simulink model "acc_aeb_top"  (R2025a)
settings: Solver=ode23t  StartTime=0.0  StopTime=40  RelTol=1e-3
undefined symbols (not defined in the file): invDiffWarnBrake, invTau_ACC, k_drag, P
libraries: sim3dautolib x2, slpidlib x1, sim3dlib x1
settings Model: Creator=harun  LastModifiedBy=harun

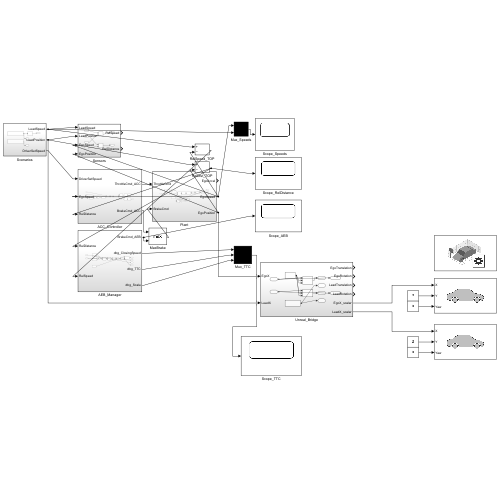
[thumbnail: Simulink's stored preview of the top-level diagram]
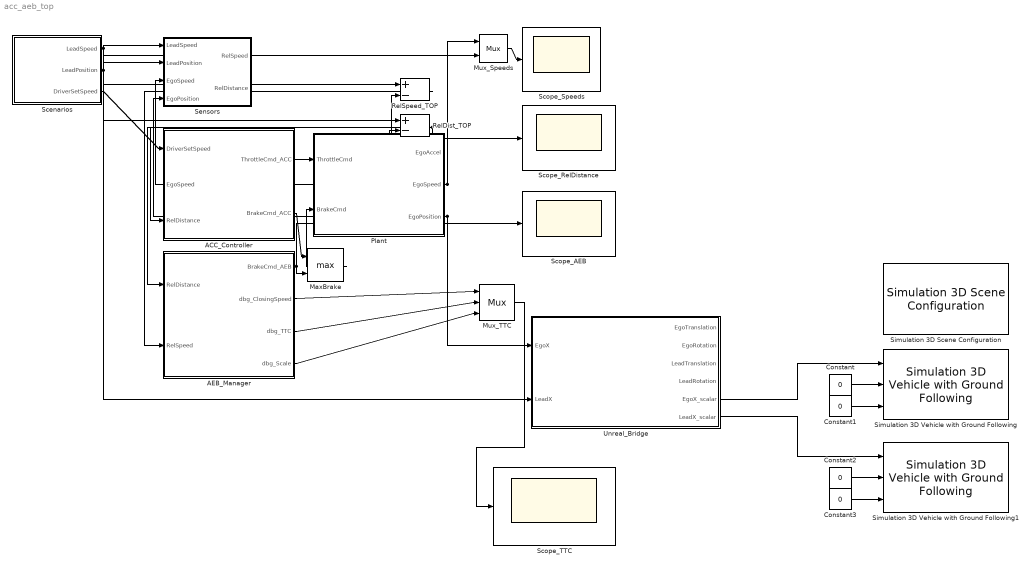
== system acc_aeb_top ==
  ACC_Controller : Subsystem
  AEB_Manager : Subsystem
  Constant{,1..3} (4 alike) : Constant  Value=0
  MaxBrake : MinMax  Function=max  Inputs=2
  Mux_Speeds : Mux  Inputs=2
  Mux_TTC : Mux  Inputs=3
  Plant : Subsystem
  RelDist_TOP : Sum  Inputs=+-
  RelSpeed_TOP : Sum  Inputs=+-
  Scenarios : Subsystem
  Scope_AEB : Scope
  Scope_RelDistance : Scope
  Scope_Speeds : Scope
  Scope_TTC : Scope
  Sensors : Subsystem
  Simulation 3D Scene Configuration : sim3dlib/Simulation 3D Scene Configuration  Priority=0  ProjectFormat=Default Scenes  SceneDesc=Straight road  ProjectName=C:\Program Files\MATLAB\R2025a\toolbox\shared\sim3d_projects\automotive_project_windows\UE\WindowsNoEditor\VehicleSimulation.exe  ScenePath=/Game/Maps/HwStrght  EnableOpenDRIVE=off  vehTagList={'Custom';'Scene Origin';'SimulinkVehicle1';'SimulinkVehicle2'}  vehTag=SimulinkVehicle1  AttachedCameraRelativeTranslation=[0 0 0]  FreeCameraDefaultInitialTranslation=[-6, 0, 2]  AttachedCameraRelativeRotation=[0 0 0]  FreeCameraDefaultInitialRotation=[0, -15, 0]  ViewpointName=Custom  FreeCameraInitialTranslation=[0, 0, 0]  ViewpointTranslation=[0 0 0]  FreeCameraInitialRotation=[0, 0, 0]  ViewpointRotation=[0 0 0]  OpVisEn=off  Ts=1/60  EnableWindow=on  EnableRemoteAccess=off  EnableWeather=off  SunAzimuth=90  SunAltitude=40.0  EnableGeospatialSun=off  Latitude=0  Longitude=0  Date=2023-01-01  Time=10:30:00  GeoTimeZone=-5.0  SunDaylightSaving=off  wind=1  clouds=10  EnableVolumetricClouds=off  CloudCoverage=0  CloudAltitude=6  fog=0  rain=0  RaindropsEffect=off  SnowDensity=0  EnableGeospatial=off  TilesetSource=Earth terrain  UseTrueOrigin=off  OriginHeight=200  OriginLatitude=40.744652  OriginLongitude=-73.988864  MapStyle=Aerial  AdditionalAssetIDs=[]  UseAdvancedSunSky=off  SolarTime=11  TimeZone=-5  Day=21  Month=9  Year=2022  UseDaylightSavingTime=on  DSTStartDay=10  DSTStartMonth=3  DSTEndDay=3  DSTEndMonth=11  DSTSwitchHour=2  sensorTag=MainCamera1  sensorId=1  sensorName=MainCamera1  mountLoc=Origin  offsetFlag=off  tmountOffset=[0, 0, 0]  rmountOffset=[0, 0, 0]  HorizontalResolution=1280  VerticalResolution=720  HorizontalFOV=60  mountPoint=[0 0 0]  mountOrientation=[0 0 0]  aMode=3  ID=1  GeoTrigger=Inactive  ViewNameList={'Custom'}  ViewTranslationList={'[0 0 0]'}  ViewRotationList={'[0 0 0]'}
      settings: LibrarySourceBlock=drivingsim3d/Simulation 3D Scene Configuration
  Simulation 3D Vehicle with Ground Following : sim3dautolib/Simulation 3D Vehicle with Ground Following  Priority=-1  PassVehMesh=Muscle car  MeshPath=/MathWorksAutomotiveContent/Vehicles/Muscle/Meshes/SK_MuscleCar.SK_MuscleCar  TrackWidth=1.9  WheelBase=3  WheelRadius=0.35  VehColor=Red  CoordinateSystem=ISO8855  InitialPos=[0, 0, 0]  InitialRot=[0, 0, 0]  ActorName=SimulinkVehicle1  SampleTime=-1  ActorType=SimulinkVehicle  ID=1  aMode=3  ActorTag=SimulinkVehicle1  CoordinateScheme=0  VehLightsControl=off  HeadlightColor=[ 1, 1, 1 ]  HighBeamIntensity=100000  LowBeamIntensity=60000  HighBeamConeAngle=70  LowBeamConeAngle=70  LeftHeadlightOrientation=[ 0, 0 ]  RightHeadlightOrientation=[ 0, 0 ]  BrakelightIntensity=500  ReverselightIntensity=500  SignallightIntensity=500  SignallightPeriod=1  SignalPulseWidth=50  TransformOutportEnabled=off
      settings: LibrarySourceBlock=drivingsim3d/Simulation 3D Vehicle with Ground Following
  Simulation 3D Vehicle with Ground Following1 : sim3dautolib/Simulation 3D Vehicle with Ground Following  Priority=-1  PassVehMesh=Muscle car  MeshPath=/MathWorksAutomotiveContent/Vehicles/Muscle/Meshes/SK_MuscleCar.SK_MuscleCar  TrackWidth=1.9  WheelBase=3  WheelRadius=0.35  VehColor=Blue  CoordinateSystem=ISO8855  InitialPos=[0, 0, 0]  InitialRot=[0, 0, 0]  ActorName=SimulinkVehicle2  SampleTime=-1  ActorType=SimulinkVehicle  ID=2  aMode=3  ActorTag=SimulinkVehicle2  CoordinateScheme=0  VehLightsControl=off  HeadlightColor=[ 1, 1, 1 ]  HighBeamIntensity=100000  LowBeamIntensity=60000  HighBeamConeAngle=70  LowBeamConeAngle=70  LeftHeadlightOrientation=[ 0, 0 ]  RightHeadlightOrientation=[ 0, 0 ]  BrakelightIntensity=500  ReverselightIntensity=500  SignallightIntensity=500  SignallightPeriod=1  SignalPulseWidth=50  TransformOutportEnabled=off
      settings: LibrarySourceBlock=drivingsim3d/Simulation 3D Vehicle with Ground Following
  Unreal_Bridge : Subsystem
  wires:
  Scenarios/1(LeadSpeed) -> Sensors/1(LeadSpeed), RelSpeed_TOP/1, Mux_Speeds/2
  Scenarios/2(LeadPosition) -> Sensors/2(LeadPosition), RelDist_TOP/1, Unreal_Bridge/2(LeadX)
  Plant/2(EgoSpeed) -> Sensors/3(EgoSpeed), ACC_Controller/2(EgoSpeed), RelSpeed_TOP/2, Mux_Speeds/1
  Plant/3(EgoPosition) -> Sensors/4(EgoPosition), RelDist_TOP/2, Unreal_Bridge/1(EgoX)
  Scenarios/3(DriverSetSpeed) -> ACC_Controller/1(DriverSetSpeed)
  RelDist_TOP/1 -> ACC_Controller/3(RelDistance), AEB_Manager/1(RelDistance), Scope_RelDistance/1
  RelSpeed_TOP/1 -> AEB_Manager/2(RelSpeed)
  ACC_Controller/2(BrakeCmd_ACC) -> MaxBrake/1
  AEB_Manager/1(BrakeCmd_AEB) -> MaxBrake/2, Scope_AEB/1
  ACC_Controller/1(ThrottleCmd_ACC) -> Plant/1(ThrottleCmd)
  MaxBrake/1 -> Plant/2(BrakeCmd)
  Mux_Speeds/1 -> Scope_Speeds/1
  AEB_Manager/2(dbg_ClosingSpeed) -> Mux_TTC/1
  AEB_Manager/3(dbg_TTC) -> Mux_TTC/2
  AEB_Manager/4(dbg_Scale) -> Mux_TTC/3
  Mux_TTC/1 -> Scope_TTC/1
  Unreal_Bridge/5(EgoX_scalar) -> Simulation 3D Vehicle with Ground Following/1
  Unreal_Bridge/6(LeadX_scalar) -> Simulation 3D Vehicle with Ground Following1/1
  Constant/1 -> Simulation 3D Vehicle with Ground Following/2
  Constant1/1 -> Simulation 3D Vehicle with Ground Following/3
  Constant2/1 -> Simulation 3D Vehicle with Ground Following1/2
  Constant3/1 -> Simulation 3D Vehicle with Ground Following1/3

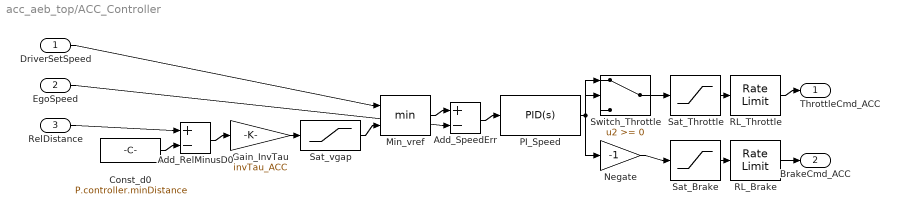
== system acc_aeb_top/ACC_Controller ==
  DriverSetSpeed : Inport
  EgoSpeed : Inport  Port=2
  RelDistance : Inport  Port=3
  Add_RelMinusD0 : Sum  Inputs=+-
  Add_SpeedErr : Sum  Inputs=+-
  Const_d0 : Constant  Value=P.controller.minDistance
  Gain_InvTau : Gain  Gain=invTau_ACC
  Min_vref : MinMax  Inputs=2
  Negate : Gain  Gain=-1
  PI_Speed : slpidlib/PID Controller  Controller=PID  Form=Parallel  TimeDomain=Continuous-time  UseExternalTs=off  SampleTime=-1  IntegratorMethod=Forward Euler  FilterMethod=Forward Euler  ControllerParametersSource=internal  P=P.controller.PI_speed.Kp  I=P.controller.PI_speed.Ki  UseKiTs=off  D=0  UseExternalDerivativeSource=off  N=100  UseFilter=on  TunerSelectOption=Transfer Function Based (PID Tuner App)  InitialConditionSource=internal  InitialConditionForIntegrator=0  InitialConditionForFilter=0  DifferentiatorICPrevScaledInput=0  ExternalReset=none  TrackingMode=off  Kt=1  LimitOutput=on  SatLimitsSource=internal  UpperSaturationLimit=P.controller.PI_speed.u_max  LowerSaturationLimit=P.controller.PI_speed.u_min  LinearizeAsGain=on  AntiWindupMode=none  Kb=1  LimitIntegrator=off  UpperIntegratorSaturationLimit=inf  LowerIntegratorSaturationLimit=-inf  POutMin=[]  POutMax=[]  IOutMin=[]  IOutMax=[]  DOutMin=[]  DOutMax=[]  NOutMin=[]  NOutMax=[]  SumOutMin=[]  SumOutMax=[]  SaturationOutMin=[]  SaturationOutMax=[]  PParamMin=[]  PParamMax=[]  IParamMin=[]  IParamMax=[]  DParamMin=[]  DParamMax=[]  NParamMin=[]  NParamMax=[]  KbParamMin=[]  KbParamMax=[]  KtParamMin=[]  KtParamMax=[]  KbOutMin=[]  KbOutMax=[]  KtOutMin=[]  KtOutMax=[]  IntegratorOutMin=[]  IntegratorOutMax=[]  FilterOutMin=[]  FilterOutMax=[]  SumI1OutMin=[]  SumI1OutMax=[]  SumI2OutMin=[]  SumI2OutMax=[]  SumI3OutMin=[]  SumI3OutMax=[]  SumI4OutMin=[]  SumI4OutMax=[]  SumDOutMin=[]  SumDOutMax=[]  DifferentiatorOutMin=[]  DifferentiatorOutMax=[]  FilterDiffOutCoefMin=[]  FilterDiffOutCoefMax=[]  ReciprocalOutMin=[]  ReciprocalOutMax=[]  SumDenOutMin=[]  SumDenOutMax=[]  SumNumOutMin=[]  SumNumOutMax=[]  DivideOutMin=[]  DivideOutMax=[]  UdiffTsProdOutMin=[]  UdiffTsProdOutMax=[]  NTsProdOutMin=[]  NTsProdOutMax=[]  UintegralTsProdOutMin=[]  UintegralTsProdOutMax=[]  UngainTsProdOutMin=[]  UngainTsProdOutMax=[]  ClampingZeroOutDataTypeStr=Inherit: Inherit via back propagation  ClampingZeroOutMin=[]  ClampingZeroOutMax=[]  FilterDenConstantOutDataTypeStr=Inherit: Inherit via back propagation  FilterDenConstantOutMin=[]  FilterDenConstantOutMax=[]  PCopyOutDataTypeStr=Inherit: Inherit via back propagation  PCopyOutMin=[]  PCopyOutMax=[]  NCopyOutDataTypeStr=Inherit: Inherit via back propagation  NCopyOutMin=[]  NCopyOutMax=[]  IntegratorContinuousStateAttributes=''  IntegratorStateMustResolveToSignalObject=off  IntegratorRTWStateStorageClass=Auto  FilterContinuousStateAttributes=''  FilterStateMustResolveToSignalObject=off  FilterRTWStateStorageClass=Auto  ParallelPVariant=InternalParameters  IdealPVariant=Disabled  IVariant=InternalParameters  DVariant=InternalParameters  IntegratorVariant=Continuous  SatVariant=Enabled  AWVariant=Passthrough  PCopyVariant=Disabled  TRVariant=Disabled  FdbkBlocksVariant=Forward  IdealPFdbkVariant=Disabled  SatFdbkVariant=Disabled  DerivativeFilterVariant=ContFilter  NVariant=InternalParameters  NCopyVariant=Disabled  FilterICVariant=InternalICsFilter  IntegratorICVariant=InternalICs  ExternalResetVariant=Disabled  TRSumVariant=Passthrough  SumFdbkVariant=Disabled  SumVariant=Sum_PID  TsampFilterVariant=InternalTs  TsampNgainVariant=Passthrough  TsampIntegralVariant=Disabled_SignalSpec  ExternalSaturationOutDataTypeStr=Inherit: Same as second input  DerivativeSourceVariant=ErrorSignal  PreIntVariant=InternalPreInt
  RL_Brake : RateLimiter  RisingSlewLimit=P.limits.rate_brake_up  FallingSlewLimit=-P.limits.rate_brake_down  SampleTimeMode=inherited
  RL_Throttle : RateLimiter  RisingSlewLimit=P.limits.rate_throttle_up  FallingSlewLimit=-P.limits.rate_throttle_down  SampleTimeMode=inherited
  Sat_Brake : Saturate  UpperLimit=0.3  LowerLimit=0
  Sat_Throttle : Saturate  UpperLimit=1  LowerLimit=0
  Sat_vgap : Saturate  UpperLimit=inf  LowerLimit=0
  Switch_Throttle : Switch  SaturateOnIntegerOverflow=off  InputSameDT=off
  ThrottleCmd_ACC : Outport
  BrakeCmd_ACC : Outport  Port=2
  wires:
  RelDistance/1 -> Add_RelMinusD0/1
  Const_d0/1 -> Add_RelMinusD0/2
  Add_RelMinusD0/1 -> Gain_InvTau/1
  Gain_InvTau/1 -> Sat_vgap/1
  DriverSetSpeed/1 -> Min_vref/1
  Sat_vgap/1 -> Min_vref/2
  Min_vref/1 -> Add_SpeedErr/1
  EgoSpeed/1 -> Add_SpeedErr/2
  Add_SpeedErr/1 -> PI_Speed/1
  PI_Speed/1 -> Switch_Throttle/1, Switch_Throttle/2, Negate/1
  Switch_Throttle/1 -> Sat_Throttle/1
  Sat_Throttle/1 -> RL_Throttle/1
  RL_Throttle/1 -> ThrottleCmd_ACC/1
  Negate/1 -> Sat_Brake/1
  Sat_Brake/1 -> RL_Brake/1
  RL_Brake/1 -> BrakeCmd_ACC/1

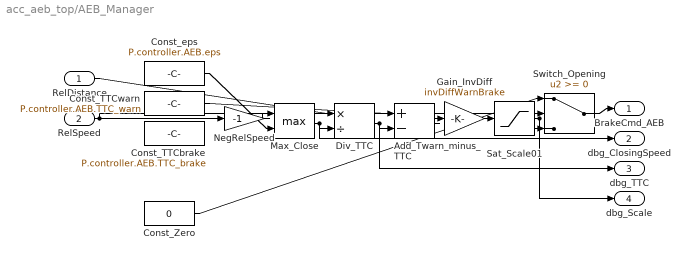
== system acc_aeb_top/AEB_Manager ==
  RelDistance : Inport
  RelSpeed : Inport  Port=2
  Add_Twarn_minus_TTC : Sum  Inputs=+-
  Const_TTCbrake : Constant  Value=P.controller.AEB.TTC_brake
  Const_TTCwarn : Constant  Value=P.controller.AEB.TTC_warn
  Const_Zero : Constant  Value=0
  Const_eps : Constant  Value=P.controller.AEB.eps
  Div_TTC : Product  Inputs=*/
  Gain_InvDiff : Gain  Gain=invDiffWarnBrake
  Max_Close : MinMax  Function=max  Inputs=2
  NegRelSpeed : Gain  Gain=-1
  Sat_Scale01 : Saturate  UpperLimit=1  LowerLimit=0
  Switch_Opening : Switch  SaturateOnIntegerOverflow=off  InputSameDT=off
  BrakeCmd_AEB : Outport
  dbg_ClosingSpeed : Outport  Port=2
  dbg_TTC : Outport  Port=3
  dbg_Scale : Outport  Port=4
  wires:
  RelSpeed/1 -> NegRelSpeed/1, Switch_Opening/2
  NegRelSpeed/1 -> Max_Close/1
  Const_eps/1 -> Max_Close/2
  RelDistance/1 -> Div_TTC/1
  Max_Close/1 -> Div_TTC/2, dbg_ClosingSpeed/1
  Const_TTCwarn/1 -> Add_Twarn_minus_TTC/1
  Div_TTC/1 -> Add_Twarn_minus_TTC/2, dbg_TTC/1
  Add_Twarn_minus_TTC/1 -> Gain_InvDiff/1
  Gain_InvDiff/1 -> Sat_Scale01/1
  Sat_Scale01/1 -> Switch_Opening/3, dbg_Scale/1
  Const_Zero/1 -> Switch_Opening/1
  Switch_Opening/1 -> BrakeCmd_AEB/1

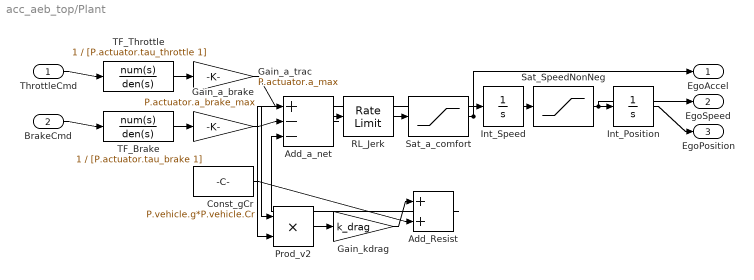
== system acc_aeb_top/Plant ==
  ThrottleCmd : Inport
  BrakeCmd : Inport  Port=2
  Add_Resist : Sum
  Add_a_net : Sum  Inputs=+--
  Const_gCr : Constant  Value=P.vehicle.g*P.vehicle.Cr
  Gain_a_brake : Gain  Gain=P.actuator.a_brake_max
  Gain_a_trac : Gain  Gain=P.actuator.a_max
  Gain_kdrag : Gain  Gain=k_drag
  Int_Position : Integrator  InitialCondition=P.scenario.ego_x0
  Int_Speed : Integrator  InitialCondition=P.scenario.ego_v0
  Prod_v2 : Product  Inputs=**
  RL_Jerk : RateLimiter  RisingSlewLimit=P.limits.jerk_limit  FallingSlewLimit=-P.limits.jerk_limit  SampleTimeMode=inherited
  Sat_SpeedNonNeg : Saturate  UpperLimit=inf  LowerLimit=0
  Sat_a_comfort : Saturate  UpperLimit=P.limits.a_comfort_pos  LowerLimit=-P.limits.a_comfort_neg
  TF_Brake : TransferFcn  Numerator=1  Denominator=[P.actuator.tau_brake 1]
  TF_Throttle : TransferFcn  Numerator=1  Denominator=[P.actuator.tau_throttle 1]
  EgoAccel : Outport
  EgoSpeed : Outport  Port=2
  EgoPosition : Outport  Port=3
  wires:
  ThrottleCmd/1 -> TF_Throttle/1
  BrakeCmd/1 -> TF_Brake/1
  TF_Throttle/1 -> Gain_a_trac/1
  TF_Brake/1 -> Gain_a_brake/1
  Gain_a_trac/1 -> Add_a_net/1
  Gain_a_brake/1 -> Add_a_net/2
  Sat_SpeedNonNeg/1 -> Prod_v2/1, Prod_v2/2, Int_Position/1, EgoSpeed/1
  Prod_v2/1 -> Gain_kdrag/1
  Gain_kdrag/1 -> Add_Resist/1
  Const_gCr/1 -> Add_Resist/2
  Add_Resist/1 -> Add_a_net/3
  Add_a_net/1 -> RL_Jerk/1
  RL_Jerk/1 -> Sat_a_comfort/1
  Sat_a_comfort/1 -> Int_Speed/1, EgoAccel/1
  Int_Speed/1 -> Sat_SpeedNonNeg/1
  Int_Position/1 -> EgoPosition/1

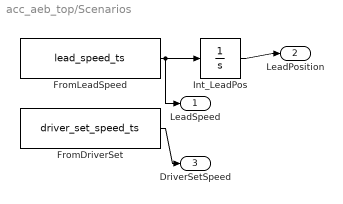
== system acc_aeb_top/Scenarios ==
  FromDriverSet : FromWorkspace  VariableName=driver_set_speed_ts
  FromLeadSpeed : FromWorkspace  VariableName=lead_speed_ts
  Int_LeadPos : Integrator  InitialCondition=P.scenario.lead_x0
  LeadSpeed : Outport
  LeadPosition : Outport  Port=2
  DriverSetSpeed : Outport  Port=3
  wires:
  FromLeadSpeed/1 -> Int_LeadPos/1, LeadSpeed/1
  Int_LeadPos/1 -> LeadPosition/1
  FromDriverSet/1 -> DriverSetSpeed/1

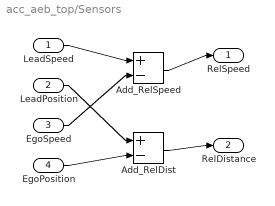
== system acc_aeb_top/Sensors ==
  LeadSpeed : Inport
  LeadPosition : Inport  Port=2
  EgoSpeed : Inport  Port=3
  EgoPosition : Inport  Port=4
  Add_RelDist : Sum  Inputs=+-
  Add_RelSpeed : Sum  Inputs=+-
  RelSpeed : Outport
  RelDistance : Outport  Port=2
  wires:
  LeadSpeed/1 -> Add_RelSpeed/1
  EgoSpeed/1 -> Add_RelSpeed/2
  LeadPosition/1 -> Add_RelDist/1
  EgoPosition/1 -> Add_RelDist/2
  Add_RelSpeed/1 -> RelSpeed/1
  Add_RelDist/1 -> RelDistance/1

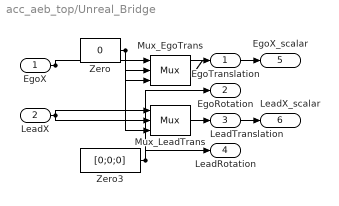
== system acc_aeb_top/Unreal_Bridge ==
  EgoX : Inport
  LeadX : Inport  Port=2
  Mux_EgoTrans : Mux  Inputs=3
  Mux_LeadTrans : Mux  Inputs=3
  Zero : Constant  Value=0
  Zero3 : Constant  Value=[0;0;0]
  EgoTranslation : Outport
  EgoRotation : Outport  Port=2
  LeadTranslation : Outport  Port=3
  LeadRotation : Outport  Port=4
  EgoX_scalar : Outport  Port=5
  LeadX_scalar : Outport  Port=6
  wires:
  EgoX/1 -> Mux_EgoTrans/1, EgoX_scalar/1
  Zero/1 -> Mux_EgoTrans/2, Mux_EgoTrans/3, Mux_LeadTrans/2, Mux_LeadTrans/3
  LeadX/1 -> Mux_LeadTrans/1, LeadX_scalar/1
  Mux_EgoTrans/1 -> EgoTranslation/1
  Mux_LeadTrans/1 -> LeadTranslation/1
  Zero3/1 -> EgoRotation/1, LeadRotation/1
